simulink subsystem "Day1_Scenario_1"  (R2024a)
settings: Solver=VariableStepAuto  StartTime=0.0  StopTime=10.0  RelTol=1e-3
libraries: CarMaker4SL x1
settings Model: Creator=junhyung.cha  LastModifiedBy=User

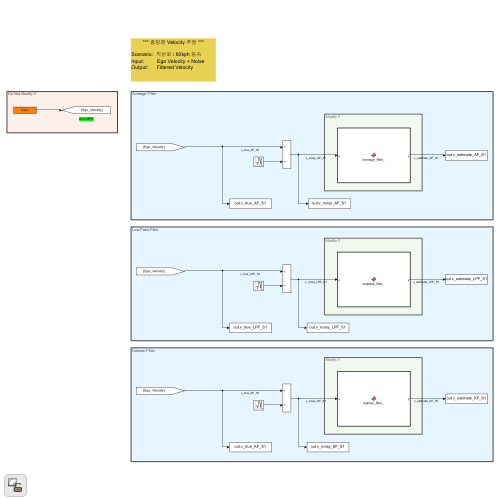
[thumbnail: Simulink's stored preview of the top-level diagram]
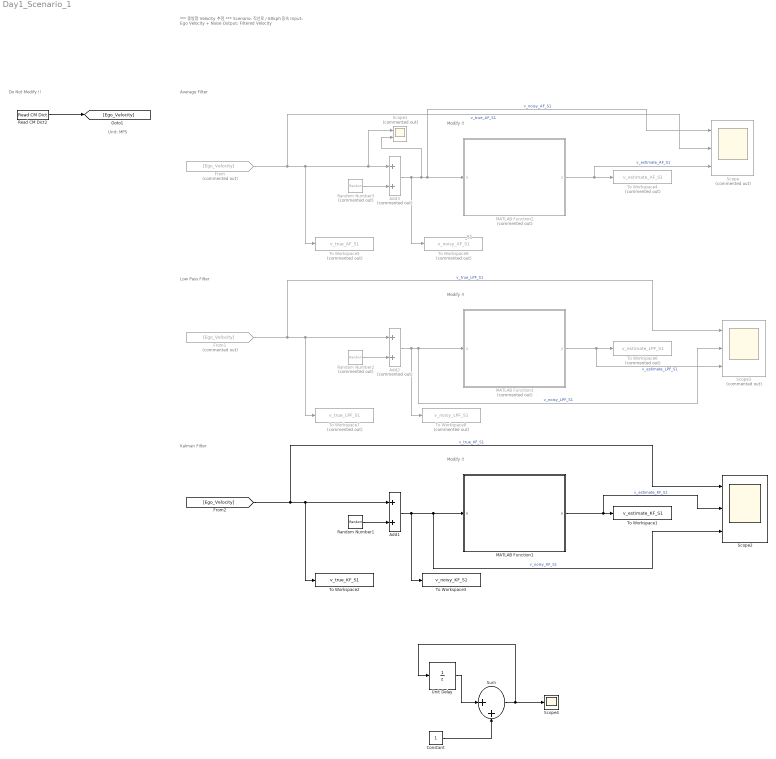
== system Day1_Scenario_1 ==
  note: _S1
  note: Modify !!
  note: Modify !!
  note: Modify !!
  note: Average Filter
  note: Low Pass Filter
  note: Kalman Filter
  note: *** 종방향 Velocity 추정 ***
      |
      | Scenario: 직선로 / 60kph 등속
      | Input: Ego Velocity + Noise
      | Output: Filtered Velocity
  note: Do Not Modify !!
  note: Unit: MPS
  Add1 : Sum
  Add2 : Sum  Commented=on
  Add3 : Sum  Commented=on
  Constant : Constant
  From : From  Commented=on  GotoTag=Ego_Velocity
  From1 : From  Commented=on  GotoTag=Ego_Velocity
  MATLAB Function1 : MATLAB Function  TreatAsAtomicUnit=on
  MATLAB Function2 : MATLAB Function  Commented=on  TreatAsAtomicUnit=on
  MATLAB Function3 : MATLAB Function  Commented=on  TreatAsAtomicUnit=on
  Random Number1 : RandomNumber
  Random Number2 : RandomNumber  Commented=on
  Random Number3 : RandomNumber  Commented=on
  Read CM Dict2 : CarMaker4SL/Read CM Dict  xname=Car.v  xsync=off  xstime=Inherited
  Scope : Scope  Commented=on  NumInputPorts=3
  Scope1 : Scope  Commented=on  NumInputPorts=2
  Scope2 : Scope  NumInputPorts=3
  Scope3 : Scope  Commented=on  NumInputPorts=3
  Scope4 : Scope
  Sum : Sum  Inputs=|++
  To Workspace1 : ToWorkspace  VariableName=v_estimate_KF_S1  SaveFormat=Timeseries  SampleTime=-1
  To Workspace2 : ToWorkspace  VariableName=v_true_KF_S1  SaveFormat=Timeseries  SampleTime=-1
  To Workspace3 : ToWorkspace  VariableName=v_noisy_KF_S1  SaveFormat=Timeseries  SampleTime=-1
  To Workspace4 : ToWorkspace  Commented=on  VariableName=v_estimate_AF_S1  SaveFormat=Timeseries  SampleTime=-1
  To Workspace5 : ToWorkspace  Commented=on  VariableName=v_true_AF_S1  SaveFormat=Timeseries  SampleTime=-1
  To Workspace6 : ToWorkspace  Commented=on  VariableName=v_estimate_LPF_S1  SaveFormat=Timeseries  SampleTime=-1
  To Workspace7 : ToWorkspace  Commented=on  VariableName=v_true_LPF_S1  SaveFormat=Timeseries  SampleTime=-1
  To Workspace8 : ToWorkspace  Commented=on  VariableName=v_noisy_LPF_S1  SaveFormat=Timeseries  SampleTime=-1
  To Workspace9 : ToWorkspace  Commented=on  VariableName=v_noisy_AF_S1  SaveFormat=Timeseries  SampleTime=-1
  Unit Delay : UnitDelay  SampleTime=-1  HasFrameUpgradeWarning=on
  wires:
  Random Number2/1 -> Add2/2
  From1/1 -> Add2/1, To Workspace7/1, Scope3/1  "v_true_LPF_S1"
  Add2/1 -> MATLAB Function3/1(u), Scope3/2, To Workspace8/1  "v_noisy_LPF_S1"
  MATLAB Function3/1(y) -> To Workspace6/1, Scope3/3  "v_estimate_LPF_S1"
  [Ego_Velocity] -> Add1/1, To Workspace2/1, Scope2/1  "v_true_KF_S1"
  MATLAB Function1/1(y) -> To Workspace1/1, Scope2/2  "v_estimate_KF_S1"
  Random Number1/1 -> Add1/2
  Add1/1 -> MATLAB Function1/1(u), Scope2/3, To Workspace3/1  "v_noisy_KF_S1"
  MATLAB Function2/1(y) -> To Workspace4/1, Scope/3  "v_estimate_AF_S1"
  Random Number3/1 -> Add3/2
  From/1 -> Add3/1, Scope1/1, To Workspace5/1, Scope/2  "v_true_AF_S1"
  Add3/1 -> MATLAB Function2/1(u), Scope/1, Scope1/2, To Workspace9/1  "v_noisy_AF_S1"
  Read CM Dict2/1 -> [Ego_Velocity]
  Unit Delay/1 -> Sum/1
  Constant/1 -> Sum/2
  Sum/1 -> Unit Delay/1, Scope4/1

== matlab function Day1_Scenario_1/MATLAB Function2 ==
  settings: updateMethod=DISCRETE  sampleTime=0.05
  data: u input; y output
% function y = average_filter_(u)
%     y = 0;
% end

function y = average_filter_(u)
% 평균 필터 (5포인트 이동 평균)
% 입력: u - 현재 noisy 값
% 출력: y - 평균 필터된 값

persistent buffer
persistent idx
persistent count

N = 15; % 평균을 낼 샘플 수 (필터 윈도우 크기)

if isempty(buffer)
    buffer = zeros(1, N);
    idx = 1;
    count = 0;
end

% 새로운 값 저장
buffer(idx) = u;
idx = idx + 1;
if idx > N
    idx = 1;
end

% 현재까지 받은 값 수 증가
if count < N
    count = count + 1;
end

% 평균 계산
y = sum(buffer) / count;

== matlab function Day1_Scenario_1/MATLAB Function3 ==
  settings: updateMethod=DISCRETE  sampleTime=0.05
  data: u input; y output
function y = lowpass_filter_(u)
% 1차 로우패스 필터
% 입력: u - 노이즈 포함된 측정값
% 출력: y - 필터링된 출력값

persistent y_prev
persistent alpha

% 필터 계수 초기화 (단 한 번만)
if isempty(y_prev)
    y_prev = 0;           % 이전 출력값 초기화
    dt = 0.001;             % 샘플링 시간 (초) - Simulink 모델과 일치시켜야 함
    tau = 0.01;            % 시정수 (필터가 얼마나 느리게 반응할지 결정)
    alpha = dt / (tau + dt);  % 로우패스 필터 계수
end

% 로우패스 필터 공식
y = alpha * u + (1 - alpha) * y_prev;

% 상태 저장
y_prev = y;

== matlab function Day1_Scenario_1/MATLAB Function1 ==
  settings: updateMethod=DISCRETE
  data: u input; y output
% function y = kalman_filter_(u)
% % 칼만 필터 (1차 상태, 샘플링 0.001초 기준)
% 
% persistent x_hat P
% persistent A H Q R
% persistent initialized
% 
% if isempty(initialized)
%     % 초기 상태
%     x_hat = 0;
%     P = 1;
% 
%     % 시스템 모델 (정지 시스템)
%     A = 1;
%     H = 1;
% 
%     % 튜닝 값
%     Q = 1e-5;  % 프로세스 노이즈: 시스템 변화가 적다면 작게
%     R = 0.1;  % 측정 노이즈: 노이즈 많으면 크게
% 
%     initialized = true;
% end
% 
% % 예측 단계
% x_hat_pred = A * x_hat;
% P_pred = A * P * A' + Q;
% 
% % 칼만 이득
% K = P_pred * H' / (H * P_pred * H' + R);
% 
% % 업데이트
% x_hat = x_hat_pred + K * (u - H * x_hat_pred);
% P = (1 - K * H) * P_pred;
% 
% % 출력
% y = x_hat;

function y = kalman_filter_(u)
% 이산 칼만 필터: 연속 시스템을 Euler 근사로 이산화한 모델 기반
% 샘플링 주기: 0.001초

persistent x_hat P
persistent A B H Q R
persistent initialized

dt = 0.001;  % 샘플링 주기

if isempty(initialized)
    % 초기 상태 추정값
    x_hat = 0;
    P = 1;

    % 연속 시스템 (예: dx/dt = a*x + b*u)
    a = -0.5;     % 상태 천이 계수 (ex: 감쇠계수 등)
    b = 1.0;      % 입력 계수

    % 이산화 (Euler 근사)
    A = 1 + a * dt;
    B = b * dt;

    % 관측 모델
    H = 1;

    % 잡음 공분산 (튜닝 파라미터)
    Q = 1e-6;  % 프로세스 노이즈 (모델 신뢰도)
    R = 0.01;   % 측정 노이즈 (센서 신뢰도)

    initialized = true;
end

% 예측 단계
x_hat_pred = A * x_hat + B * u;
P_pred = A * P * A' + Q;

% 칼만 이득 계산
K = P_pred * H' / (H * P_pred * H' + R);

% 상태 추정값 업데이트
x_hat = x_hat_pred + K * (u - H * x_hat_pred);
P = (1 - K * H) * P_pred;

% 결과 출력
y = x_hat;
